simulink model "x35BusNetworkElectricityTransmissionModel"  (R2023b)
settings: Solver=VariableStepAuto  StartTime=0.0  StopTime=0.8  RelTol=1e-3
model workspace (MAT data in the model file):
  Compensation_Ki = 30
  Compensation_Kp = 3
  DC_Ki = 400
  DC_Kp = 8
  F = 0.01
  Flux_min = 0.5
  Grid_Freq_PWM = 2700
  Grid_Ireg_Ki = 5
  Grid_Ireg_Kp = 0.83
  Grid_Ireg_lim = 1.1
  Grid_Modindex_Upper = 1.1
  Grid_conv_Imax = 0.8
  H = 0.685
  Idref_max = 0.9
  Iqref_Tc = 0.3
  Ki_Var = 0.05
  Ki_Vreg = 20
  Ksh = 1.1
  L_pu = 0.3
  Llr = 0.16
  Lls = 0.18
  Lm = 2.9
  Nb_wt = 6
  P_mech = 1080000
  Pitch_Ki = 0
  Pitch_Kp = 150
  Pitch_Max = 27
  Pitch_Tc = 0.01
  Pitch_rate = 10
  Q_Filt = 50
  R_pu = 0.003
  Rotor_Freq_PWM = 1620
  Rotor_Ireg_Ki = 8
  Rotor_Ireg_Kp = 0.6
  Rotor_Ireg_lim = 0.1
  Rotor_Modindex_Upper = 2
  Rr = 0.016
  Rs = 0.023
  T_set = 0.0001
  Tp = 5e-05
  Ts = 5e-06
  Var_C_Filt = 720000
  Var_reg_max = 1.1
  Var_reg_min = 0.9
  WT_Coeff = [0.645 116 0.4 5 21 0.00912 0.08 0.035]
  WT_H = 4.32
  WT_IGBTRon = 5.931
  WT_Param = [91.204 10143]
  Wind_Freq_Filt = 10000
  Wind_Freq_nom = 60
  Wind_P_nom = 1200000
  Wind_Rotor_V_nom = 1950
  Wind_V_nom = 500
  Zeta_Filt = 0.707106781187
  init = [-0.2 0 0 0 0 0 0 0]
  p = 3
  torque0 = 0.83
  v_Ki = 0.1
  v_Kp = 3.6
  v_Max = 1.2
  v_Min = 0.7
  v_T = 5
  vreg_max = 1
  wind_VDC_nom = 1150
  wt0 = 1.2
undefined symbols (not defined in the file): D1, D11, Delta, DiscIntNeverNeededParam, Ion, Lithium, P, Q
libraries: powerlib_extras x144, spsSeriesRLCBranchLib x67, spsLoadFlowBusLib x43, spsThreePhaseTransformerTwoWindingsLib x32, spsThreePhaseSeriesRLCLoadLib x31, spsThreePhaseVIMeasurementLib x26, simulink_extras x26, spsDistributedParametersLineLib x22, spsGenericPowerSystemStabilizerLib x20, spsSynchronousMachinepuStandardLib x10, spsExcitationSystemLib x10, spsHydraulicTurbineandGovernorLib x10
(part 2 of 16)

== system x35BusNetworkElectricityTransmissionModel/ 41.4 MW Wind Generation ==
  " 64 MVA 115KV :20KV Transformer " : spsThreePhaseTransformerTwoWindingsLib/Three-Phase Transformer (Two Windings)  Winding1Connection=Yg  Winding2Connection=Delta (D1)  CoreType=Three single-phase transformers  SetSaturation=off  Hysteresis=off  DataFile='hysteresis'  SetInitialFlux=off  Measurements=None  UNITS=pu  NominalPower=[ 64e6 , 60 ]  Winding1=[ 115e3 , 0.002 , 0.08 ]  Winding2=[ 20e3 , 0.002 , 0.08 ]  Rm=500  Lm=500  L0=0.5  Saturation=[ 0,0 ; 0.0024,1.2 ; 1.0,1.52 ]  InitialFluxes=[ 0.8 , -0.8 , 0.7 ]  BreakLoop=off  DiscreteSolver=Trapezoidal iterative  DataType=off  TransfoNumber=1
  " Tie to Ground Transformer " : spsThreePhaseTransformerTwoWindingsLib/Three-Phase Transformer (Two Windings)  Winding1Connection=Yn  Winding2Connection=Delta (D11)  CoreType=Three single-phase transformers  SetSaturation=off  Hysteresis=off  DataFile='hysteresis'  SetInitialFlux=off  Measurements=None  UNITS=pu  NominalPower=[ 5600e6 , 60 ]  Winding1=[ 13.8e3 , 0.002 , 0.08 ]  Winding2=[ 735e3 , 0.002 , 0.08 ]  Rm=500  Lm=500  L0=0.5  Saturation=[ 0,0 ; 0.0024,1.2 ; 1.0,1.52 ]  InitialFluxes=[ 0.8 , -0.8 , 0.7 ]  BreakLoop=off  DiscreteSolver=Trapezoidal iterative  DataType=off  TransfoNumber=1
  150 kVar : spsThreePhaseSeriesRLCLoadLib/Three-Phase Series RLC Load  LConnTagsString=A|B|C  Configuration=Y (grounded)  NominalVoltage=20e3  Vabc=[1e3 1e3 1e3]  Vabcp=[1e3 1e3 1e3]  NominalFrequency=60  UnbalancedPower=off  ActivePower=0  InductivePower=0  CapacitivePower=150e3  Pabc=[10e3 9e3 11e3]  QLabc=[100 90 110]  QCabc=[100 90 110]  Pabcp=[10e3 9e3 11e3]  QLabcp=[100 90 110]  QCabcp=[100 90 110]  Measurements=None  LoadType=constant Z
  3.3MVar : spsThreePhaseSeriesRLCLoadLib/Three-Phase Series RLC Load  LConnTagsString=A|B|C  Configuration=Y (grounded)  NominalVoltage=20e3  Vabc=[1e3 1e3 1e3]  Vabcp=[1e3 1e3 1e3]  NominalFrequency=60  UnbalancedPower=off  ActivePower=0  InductivePower=0  CapacitivePower=3.3e6  Pabc=[10e3 9e3 11e3]  QLabc=[100 90 110]  QCabc=[100 90 110]  Pabcp=[10e3 9e3 11e3]  QLabcp=[100 90 110]  QCabcp=[100 90 110]  Measurements=None  LoadType=constant Z
  38 km : spsThreePhasePISectionLineLib/Three-Phase PI Section Line  LConnTagsString=a|b|c  RConnTagsString=A|B|C  Length=38  Frequency=60  Resistances=[ 0.01273 0.3864]/6  Inductances="[ 0.9337e-3  4.1264e-3]/6"  Capacitances=[12.74e-9 7.751e-9]*6
  41.4 MW Wind Farm : Subsystem
  4200 MW : spsThreePhaseParallelRLCLoadLib/Three-Phase Parallel RLC Load  LConnTagsString=A|B|C  Configuration=Y (grounded)  NominalVoltage=115e3  Vabc=[1e3 1e3 1e3]  Vabcp=[1e3 1e3 1e3]  NominalFrequency=60  UnbalancedPower=off  ActivePower=4200e6  InductivePower=0  CapacitivePower=0  Pabc=[10e3 9e3 11e3]  QLabc=[100 90 110]  QCabc=[100 90 110]  Pabcp=[10e3 9e3 11e3]  QLabcp=[100 90 110]  QCabcp=[100 90 110]  Measurements=None  LoadType=constant Z
  "4700 MVA 650KV :115KV Transformer " : spsThreePhaseTransformerTwoWindingsLib/Three-Phase Transformer (Two Windings)  Winding1Connection=Yg  Winding2Connection=Delta (D1)  CoreType=Three single-phase transformers  SetSaturation=off  Hysteresis=off  DataFile='hysteresis'  SetInitialFlux=off  Measurements=None  UNITS=pu  NominalPower=[ 4700e6 , 60 ]  Winding1=[ 650e3 , 0.002 , 0.08 ]  Winding2=[ 115e3 , 0.002 , 0.08 ]  Rm=500  Lm=500  L0=0.5  Saturation=[ 0,0 ; 0.0024,1.2 ; 1.0,1.52 ]  InitialFluxes=[ 0.8 , -0.8 , 0.7 ]  BreakLoop=off  DiscreteSolver=Trapezoidal iterative  DataType=off  TransfoNumber=1
  B2 : spsThreePhaseVIMeasurementLib/Three-Phase V-I Measurement  VoltageMeasurement=no  SetLabelV=off  LabelV=Vabc  Vpu=off  VpuLL=off  CurrentMeasurement=no  SetLabelI=off  LabelI=Iabc  Ipu=off  Pbase=100e6  Vbase=500e3  OutputType=Complex  PhasorSimulation=off  PSBequivalent=0
  Ground : spsGroundLib/Ground  LConnTagsString=a
  Load Flow Bus2 : spsLoadFlowBusLib/Load Flow Bus  LConnTagsString=a  Phases=single  Connectors=on one side  ID=BUS_28  Vbase=115e3  Vref=1  Vangle=0  VLF=1  VLFb=1  VLFc=1  angleLF=0  angleLFb=0  angleLFc=0
  Load Flow Bus7 : spsLoadFlowBusLib/Load Flow Bus  LConnTagsString=a  Phases=single  Connectors=on one side  ID=BUS_29  Vbase=20e3  Vref=1  Vangle=0  VLF=1  VLFb=1  VLFc=1  angleLF=0  angleLFb=0  angleLFc=0
  Series RLC Branch : spsSeriesRLCBranchLib/Series RLC Branch  LConnTagsString=__new0  RConnTagsString=__new0  BranchType=R  Resistance=4.1  Inductance=0  SetiL0=off  InitialCurrent=0  Capacitance=0  Setx0=off  InitialVoltage=0  Measurements=None
  A : PMIOPort  Side=Left
  B : PMIOPort  Port=2  Side=Left
  C : PMIOPort  Port=3  Side=Left
  connections:
  " Tie to Ground Transformer "/LConn4 -- Series RLC Branch/LConn1
  "4700 MVA 650KV :115KV Transformer "/RConn1 -- " 64 MVA 115KV :20KV Transformer "/LConn1 -- Load Flow Bus2/LConn1 -- 4200 MW/LConn1
  "4700 MVA 650KV :115KV Transformer "/RConn2 -- " 64 MVA 115KV :20KV Transformer "/LConn2 -- 4200 MW/LConn2
  "4700 MVA 650KV :115KV Transformer "/RConn3 -- " 64 MVA 115KV :20KV Transformer "/LConn3 -- 4200 MW/LConn3
  38 km/LConn2 -- " Tie to Ground Transformer "/LConn2 -- " 64 MVA 115KV :20KV Transformer "/RConn2 -- 3.3MVar/LConn2
  38 km/LConn3 -- " Tie to Ground Transformer "/LConn3 -- " 64 MVA 115KV :20KV Transformer "/RConn3 -- 3.3MVar/LConn3
  38 km/LConn1 -- " Tie to Ground Transformer "/LConn1 -- " 64 MVA 115KV :20KV Transformer "/RConn1 -- 3.3MVar/LConn1 -- Load Flow Bus7/LConn1
  Series RLC Branch/RConn1 -- Ground/LConn1
  "4700 MVA 650KV :115KV Transformer "/LConn1 -- A/RConn1
  "4700 MVA 650KV :115KV Transformer "/LConn3 -- C/RConn1
  "4700 MVA 650KV :115KV Transformer "/LConn2 -- B/RConn1
  150 kVar/LConn1 -- 38 km/RConn1 -- B2/RConn1
  B2/RConn3 -- 38 km/RConn3 -- 150 kVar/LConn3
  B2/RConn2 -- 38 km/RConn2 -- 150 kVar/LConn2
  41.4 MW Wind Farm/LConn1 -- B2/LConn1
  41.4 MW Wind Farm/LConn2 -- B2/LConn2
  41.4 MW Wind Farm/LConn3 -- B2/LConn3

== system x35BusNetworkElectricityTransmissionModel/400 kV Solar Farm ==
  3-Level Bridge : spsThreeLevelBridgeLib/Three-Level Bridge  Arms=3  SnubberResistance=1e6  SbubberCapacitance=inf  Device=IGBT / Diodes  Ron=0.2e-3  ForwardVoltages="[  0  0 ]"  Measurements=None
      settings: AttributesFormatString=\n
  "400 kVA 260V :25 kV Transformer " : spsThreePhaseTransformerTwoWindingsLib/Three-Phase Transformer (Two Windings)  Winding1Connection=Delta (D1)  Winding2Connection=Yg  CoreType=Three single-phase transformers  SetSaturation=off  Hysteresis=off  DataFile='hysteresis'  SetInitialFlux=off  Measurements=None  UNITS=pu  NominalPower=[ 400e3 , 60 ]  Winding1=[ 260 , 0.002 , 0.08 ]  Winding2=[ 25e3 , 0.002 , 0.08 ]  Rm=500  Lm=500  L0=0.5  Saturation=[ 0,0 ; 0.0024,1.2 ; 1.0,1.52 ]  InitialFluxes=[ 0.8 , -0.8 , 0.7 ]  BreakLoop=off  DiscreteSolver=Trapezoidal iterative  DataType=off  TransfoNumber=1
  "50 MVA 25kV :150 kV Transformer " : spsThreePhaseTransformerTwoWindingsLib/Three-Phase Transformer (Two Windings)  Winding1Connection=Delta (D1)  Winding2Connection=Yg  CoreType=Three single-phase transformers  SetSaturation=off  Hysteresis=off  DataFile='hysteresis'  SetInitialFlux=off  Measurements=None  UNITS=pu  NominalPower=[ 50e6 , 60 ]  Winding1=[ 25e3 , 0.002 , 0.08 ]  Winding2=[ 150e3 , 0.002 , 0.08 ]  Rm=500  Lm=500  L0=0.5  Saturation=[ 0,0 ; 0.0024,1.2 ; 1.0,1.52 ]  InitialFluxes=[ 0.8 , -0.8 , 0.7 ]  BreakLoop=off  DiscreteSolver=Trapezoidal iterative  DataType=off  TransfoNumber=1
  8000 MVA 150kV :650 kV Transformer 1 : spsThreePhaseTransformerTwoWindingsLib/Three-Phase Transformer (Two Windings)  Winding1Connection=Delta (D1)  Winding2Connection=Yg  CoreType=Three single-phase transformers  SetSaturation=off  Hysteresis=off  DataFile='hysteresis'  SetInitialFlux=off  Measurements=None  UNITS=pu  NominalPower=[8000e6 , 60 ]  Winding1=[ 150e3 , 0.002 , 0.08 ]  Winding2=[ 650e3 , 0.002 , 0.08 ]  Rm=500  Lm=500  L0=0.5  Saturation=[ 0,0 ; 0.0024,1.2 ; 1.0,1.52 ]  InitialFluxes=[ 0.8 , -0.8 , 0.7 ]  BreakLoop=off  DiscreteSolver=Trapezoidal iterative  DataType=off  TransfoNumber=1
  DC/DC Boost Converter : Subsystem
  DC/DC Boost Converter1 : Subsystem
  DC/DC Boost Converter2 : Subsystem
  DC/DC Boost Converter3 : Subsystem
  Deblock Converter : Step  Time=0.02  SampleTime=0
  Irradiance{,1..2,4} (4 alike) : eeStairGenerator/Stair Generator  LabelModeActiveChoice=Discrete  TimeInput=[0, 0.3, 0.5]  AmplitudeInput=[1000 100 1000]  SampleTime=Tp  RepeatPattern=off  OutDataTypeStr=double
      settings: LibrarySourceBlock=ee_sl_lib/General Control/Stair Generator
  Load Flow Bus1 : spsLoadFlowBusLib/Load Flow Bus  LConnTagsString=a  Phases=single  Connectors=on one side  ID=BUS_39  Vbase=25e3  Vref=1  Vangle=0  VLF=1  VLFb=1  VLFc=1  angleLF=0  angleLFb=0  angleLFc=0
  Load Flow Bus2 : spsLoadFlowBusLib/Load Flow Bus  LConnTagsString=a  Phases=single  Connectors=on one side  ID=BUS_40  Vbase=260  Vref=1  Vangle=0  VLF=1  VLFb=1  VLFc=1  angleLF=0  angleLFb=0  angleLFc=0
  Load Flow Bus6 : spsLoadFlowBusLib/Load Flow Bus  LConnTagsString=a  Phases=single  Connectors=on one side  ID=BUS_38  Vbase=150e3  Vref=1  Vangle=0  VLF=1  VLFb=1  VLFc=1  angleLF=0  angleLFb=0  angleLFc=0
  PV Array{,1..3} (4 alike) : spsPVArrayLib/PV Array  Npar=64  Nser=5  PlotType=array @ 1000 W/m2 & specified temperatures  S_vec="[ 1000  500  100 ]"  Temp_C_vec="[ 45 25  ]"  ModuleName=SunPower SPR-315E-WHT-D  PlotWhenSelected=off  Pm=315.072  Ncell=96  Voc=64.6  Isc=6.14  Vm=54.7  Im=5.76  beta_Voc_pc=-0.2727  alpha_Isc_pc=0.061743  beta_Voc=-0.17616  alpha_Isc=0.003791  IL=6.1461  I0=6.5067e-12  nI=0.95071  Rsh=430.0666  Rs=0.43041  RobustModel=on  RobustCellTemperature=45  BAL=on  Tc=1e-6  Tfilter=5e-5
  Product1 : Product
  Rate Limiter{,1..3} (4 alike) : RateLimiter  RisingSlewLimit=8000  FallingSlewLimit=-8000  SampleTimeMode=inherited  InitialCondition=1000
  Series RLC Branch1 : spsSeriesRLCBranchLib/Series RLC Branch  LConnTagsString=__new0  RConnTagsString=__new0  BranchType=C  Resistance=1  Inductance=1e-3  SetiL0=off  InitialCurrent=0  Capacitance=0.012  Setx0=off  InitialVoltage=250  Measurements=None
  Series RLC Branch2 : spsSeriesRLCBranchLib/Series RLC Branch  LConnTagsString=__new0  RConnTagsString=__new0  BranchType=C  Resistance=1  Inductance=1e-3  SetiL0=off  InitialCurrent=0  Capacitance=0.012  Setx0=off  InitialVoltage=250  Measurements=None
  Three-Phase Series RLC Branch : spsThreePhaseSeriesRLCBranchLib/Three-Phase Series RLC Branch  LConnTagsString=A|B|C  RConnTagsString=A|B|C  BranchType=RL  Resistance=1.2e-3  Inductance=45e-6  Capacitance=1e-6  Measurements=None
  Three-Phase Series RLC Load : spsThreePhaseSeriesRLCLoadLib/Three-Phase Series RLC Load  LConnTagsString=A|B|C  Configuration=Y (grounded)  NominalVoltage=260  Vabc=[1e3 1e3 1e3]  Vabcp=[1e3 1e3 1e3]  NominalFrequency=60  UnbalancedPower=off  ActivePower=41e3  InductivePower=0  CapacitivePower=41e3  Pabc=[10e3 9e3 11e3]  QLabc=[100 90 110]  QCabc=[100 90 110]  Pabcp=[10e3 9e3 11e3]  QLabcp=[100 90 110]  QCabcp=[100 90 110]  Measurements=None  LoadType=constant Z
  Three-Phase V-I Measurement1 : spsThreePhaseVIMeasurementLib/Three-Phase V-I Measurement  VoltageMeasurement=phase-to-ground  SetLabelV=on  LabelV=V_grid  Vpu=off  VpuLL=off  CurrentMeasurement=yes  SetLabelI=on  LabelI=I_grid  Ipu=off  Pbase=100e6  Vbase=500e3  OutputType=Complex  PhasorSimulation=off  PSBequivalent=0
  VSC Control : Subsystem  mask(VSC Main Controller){nom=[ 400e3  60 ], Vnom=[ 25e3 260 ], Vnom_dc=500, RLxfo=[0.002  0.06 ], RLchoke=[1e-3  45e-6  ], K_VDCreg=[7  800], K_Ireg=[0.3 20], Ts=T_set}
      mask prompts: nom "Nominal power and frequency [ Pnom(VA)  Fnom(Hz) ]:"; Vnom "Nominal primary and secondary voltages (Vrms LL) [ Vnom_prim   Vnom_sec ]:"; Vnom_dc "Nominal DC bus voltage (V):"; RLxfo "Total transformer leakage impedance (pu/Pnom) [ Rxfo  Lxf ]"; RLchoke "Choke impedance [ R(ohm) L(H) ]"; K_VDCreg "VDC regultator gains [ Kp  Ki ]:"; K_Ireg "Current regulator gains [ Kp  Ki ]:"; Ts "Sample time"
      mask init:
      | Pnom=nom(1);
      | Fnom=nom(2);
      | Vnom_prim=Vnom(1);
      | Vnom_sec=Vnom(2);
      | Zbase=Vnom_sec^2/Pnom;
      | Rtot_pu=RLxfo(1) + RLchoke(1)/Zbase;
      | Ltot_pu=RLxfo(2) + RLchoke(2)/(Zbase/(2*pi*Fnom));
      | Kp_VDCreg=K_VDCreg(1);
      | Ki_VDCreg=K_VDCreg(2);
      | Kp_Ireg=K_Ireg(1);
      | Ki_Ireg=K_Ireg(2);
      | Vdc_ref=Vnom_dc;
      | % Used to determine initial value of Boost Control (MPPT)
      | assignin('base','Vdc_ref_Inv',Vdc_ref);
  Voltage Measurement1 : spsVoltageMeasurementLib/Voltage Measurement  PhasorSimulation=off  OutputType=Complex  PSBequivalent=0
  A : PMIOPort  Side=Left
  "B " : PMIOPort  Port=2  Side=Left
  C : PMIOPort  Port=3  Side=Left
  wires:
  PV Array/1 -> DC/DC Boost Converter/1(m)
  Irradiance/1 -> Rate Limiter/1
  VSC Control/1(Pulses) -> Product1/2
  Product1/1 -> 3-Level Bridge/1
  Voltage Measurement1/1 -> [V_DC]
  [V_DC] -> VSC Control/3(Vdc_mes)
  [V_grid] -> VSC Control/1(Vabc_prim)
  [I_grid] -> VSC Control/2(Iabc_prim)
  PV Array1/1 -> DC/DC Boost Converter1/1(m)
  Irradiance4/1 -> Rate Limiter1/1
  PV Array2/1 -> DC/DC Boost Converter2/1(m)
  Irradiance1/1 -> Rate Limiter2/1
  Deblock Converter/1 -> Product1/1
  PV Array3/1 -> DC/DC Boost Converter3/1(m)
  Irradiance2/1 -> Rate Limiter3/1
  Rate Limiter/1 -> PV Array/1
  Rate Limiter1/1 -> PV Array1/1
  Rate Limiter2/1 -> PV Array2/1
  Rate Limiter3/1 -> PV Array3/1
  connections:
  Three-Phase Series RLC Load/LConn1 -- Three-Phase Series RLC Branch/RConn1 -- Load Flow Bus2/LConn1 -- "400 kVA 260V :25 kV Transformer "/LConn1
  Three-Phase Series RLC Load/LConn2 -- Three-Phase Series RLC Branch/RConn2 -- "400 kVA 260V :25 kV Transformer "/LConn2
  Three-Phase Series RLC Load/LConn3 -- Three-Phase Series RLC Branch/RConn3 -- "400 kVA 260V :25 kV Transformer "/LConn3
  8000 MVA 150kV :650 kV Transformer 1/LConn1 -- "50 MVA 25kV :150 kV Transformer "/RConn1 -- Load Flow Bus6/LConn1
  8000 MVA 150kV :650 kV Transformer 1/LConn2 -- "50 MVA 25kV :150 kV Transformer "/RConn2
  "50 MVA 25kV :150 kV Transformer "/RConn3 -- 8000 MVA 150kV :650 kV Transformer 1/LConn3
  A/RConn1 -- 8000 MVA 150kV :650 kV Transformer 1/RConn1
  "B "/RConn1 -- 8000 MVA 150kV :650 kV Transformer 1/RConn2
  C/RConn1 -- 8000 MVA 150kV :650 kV Transformer 1/RConn3
  Three-Phase Series RLC Branch/LConn1 -- 3-Level Bridge/LConn1
  Three-Phase Series RLC Branch/LConn2 -- 3-Level Bridge/LConn2
  Three-Phase Series RLC Branch/LConn3 -- 3-Level Bridge/LConn3
  DC/DC Boost Converter/LConn1 -- PV Array/RConn1
  DC/DC Boost Converter/LConn2 -- PV Array/RConn2
  DC/DC Boost Converter1/LConn2 -- PV Array1/RConn2
  DC/DC Boost Converter1/LConn1 -- PV Array1/RConn1
  DC/DC Boost Converter2/LConn2 -- PV Array2/RConn2
  DC/DC Boost Converter2/LConn1 -- PV Array2/RConn1
  Series RLC Branch1/RConn1 -- Series RLC Branch2/LConn1 -- 3-Level Bridge/RConn2
  DC/DC Boost Converter/RConn1 -- Voltage Measurement1/LConn1 -- 3-Level Bridge/RConn1 -- Series RLC Branch1/LConn1 -- DC/DC Boost Converter1/RConn1 -- DC/DC Boost Converter3/RConn1 -- DC/DC Boost Converter2/RConn1
  DC/DC Boost Converter/RConn2 -- DC/DC Boost Converter1/RConn2 -- 3-Level Bridge/RConn3 -- Voltage Measurement1/LConn2 -- Series RLC Branch2/RConn1 -- DC/DC Boost Converter3/RConn2 -- DC/DC Boost Converter2/RConn2
  DC/DC Boost Converter3/LConn1 -- PV Array3/RConn1
  DC/DC Boost Converter3/LConn2 -- PV Array3/RConn2
  Three-Phase V-I Measurement1/LConn1 -- "400 kVA 260V :25 kV Transformer "/RConn1
  Three-Phase V-I Measurement1/LConn2 -- "400 kVA 260V :25 kV Transformer "/RConn2
  Three-Phase V-I Measurement1/LConn3 -- "400 kVA 260V :25 kV Transformer "/RConn3
  Three-Phase V-I Measurement1/RConn3 -- "50 MVA 25kV :150 kV Transformer "/LConn3
  Three-Phase V-I Measurement1/RConn2 -- "50 MVA 25kV :150 kV Transformer "/LConn2
  Three-Phase V-I Measurement1/RConn1 -- "50 MVA 25kV :150 kV Transformer "/LConn1 -- Load Flow Bus1/LConn1

== system x35BusNetworkElectricityTransmissionModel/BESS ==
  "45 MVA 20kV :250 kV Transformer " : spsThreePhaseTransformerTwoWindingsLib/Three-Phase Transformer (Two Windings)  Winding1Connection=Delta (D1)  Winding2Connection=Yg  CoreType=Three single-phase transformers  SetSaturation=off  Hysteresis=off  DataFile='hysteresis'  SetInitialFlux=off  Measurements=None  UNITS=pu  NominalPower=[ 45e6 , 60 ]  Winding1=[ 20e3 , 0.002 , 0.08 ]  Winding2=[ 250e3 , 0.002 , 0.08 ]  Rm=500  Lm=500  L0=0.5  Saturation=[ 0,0 ; 0.0024,1.2 ; 1.0,1.52 ]  InitialFluxes=[ 0.8 , -0.8 , 0.7 ]  BreakLoop=off  DiscreteSolver=Trapezoidal iterative  DataType=off  TransfoNumber=1
  "450 kVA 250 V :20 kV Transformer " : spsThreePhaseTransformerTwoWindingsLib/Three-Phase Transformer (Two Windings)  Winding1Connection=Delta (D1)  Winding2Connection=Yg  CoreType=Three single-phase transformers  SetSaturation=off  Hysteresis=off  DataFile='hysteresis'  SetInitialFlux=off  Measurements=None  UNITS=pu  NominalPower=[ 450e3 , 60 ]  Winding1=[ 250 , 0.002 , 0.08 ]  Winding2=[ 20e3 , 0.002 , 0.08 ]  Rm=500  Lm=500  L0=0.5  Saturation=[ 0,0 ; 0.0024,1.2 ; 1.0,1.52 ]  InitialFluxes=[ 0.8 , -0.8 , 0.7 ]  BreakLoop=off  DiscreteSolver=Trapezoidal iterative  DataType=off  TransfoNumber=1
  "5000 MVA 250kV :650 kV Transformer " : spsThreePhaseTransformerTwoWindingsLib/Three-Phase Transformer (Two Windings)  Winding1Connection=Delta (D1)  Winding2Connection=Yg  CoreType=Three single-phase transformers  SetSaturation=off  Hysteresis=off  DataFile='hysteresis'  SetInitialFlux=off  Measurements=None  UNITS=pu  NominalPower=[ 5000e6 , 60 ]  Winding1=[ 250e3 , 0.002 , 0.08 ]  Winding2=[ 650e3 , 0.002 , 0.08 ]  Rm=500  Lm=500  L0=0.5  Saturation=[ 0,0 ; 0.0024,1.2 ; 1.0,1.52 ]  InitialFluxes=[ 0.8 , -0.8 , 0.7 ]  BreakLoop=off  DiscreteSolver=Trapezoidal iterative  DataType=off  TransfoNumber=1
  Battery Management System : Subsystem
  Battery2 : spsBatteryLib/Battery  BatType=Lithium-Ion  ShowTempParam=off  ThermalPreset=no  ShowAgeParam=off  NomV=250  NomQ=3e5  SOC=95  Batt_Tr=30  PresetModel=on  MaxQ=300000  MinV=187.5  FullV=290.9968  Dis_rate=130434.7826  R=8.3333e-06  Normal_OP=271304.3478  expZone="[270.096463      14739.1304]"  current=[6.5 13 32.5]  Units=Time  Tci=20  NomT=20  T2=-30  MaxQ2=4.8  FullV2=7.1  Normal_OP2=5.655  expZone2="[6.58           1]"  Rca=0.6  ti=2000  Dp=0  Neq0=0  Tsim=1e6  Ta1=25  Qeol=5.4*0.9  Reol=0.013333*1.2  Char_age=[2.3478, 3]  Dis_age=[2.3478, 10]  N1=1500  N2=10500  N3=1000  N4=1400  Ta2=45  N5=950
  Bus Selector : BusSelector  OutputSignals=SOC (%),Current (A),Voltage (V)
  IGBT/Diode : spsIGBTDiodeLib/IGBT//Diode  Ron=1e-3  Rs=1e5  Cs=inf  Measurements=on
  IGBT/Diode1 : spsIGBTDiodeLib/IGBT//Diode  Ron=1e-3  Rs=1e5  Cs=inf  Measurements=on
  Power Calculation : Subsystem
  Series RLC Branch : spsSeriesRLCBranchLib/Series RLC Branch  LConnTagsString=__new0  RConnTagsString=__new0  BranchType=L  Resistance=0  Inductance=2e-3  SetiL0=off  InitialCurrent=0  Capacitance=0  Setx0=off  InitialVoltage=0  Measurements=None
  Series RLC Branch3 : spsSeriesRLCBranchLib/Series RLC Branch  LConnTagsString=__new0  RConnTagsString=__new0  BranchType=RL  Resistance=0.058  Inductance=20  SetiL0=off  InitialCurrent=0  Capacitance=1e-6  Setx0=off  InitialVoltage=0  Measurements=None
  Series RLC Branch4 : spsSeriesRLCBranchLib/Series RLC Branch  LConnTagsString=__new0  RConnTagsString=__new0  BranchType=R  Resistance=2  Inductance=20  SetiL0=off  InitialCurrent=0  Capacitance=1e-6  Setx0=off  InitialVoltage=0  Measurements=None
  Terminator : Terminator
  Terminator1 : Terminator
  Three-Phase Breaker : spsThreePhaseBreakerLib/Three-Phase Breaker  InitialState=open  SwitchA=on  SwitchB=on  SwitchC=on  SwitchTimes="[0.2  0.5]"  External=off  BreakerResistance=0.01  SnubberResistance=1e6  SnubberCapacitance=inf  Measurements=None
  Universal Bridge : spsUniversalBridgeLib/Universal Bridge  Arms=3  SnubberResistance=1e5  SnubberCapacitance=inf  Device=Diodes  Ron=1e-3  Lon=0  ForwardVoltages="[  0  0  ]"  ForwardVoltage=0  GTOparameters=[ 10e-6 , 20e-6 ]  IGBTparameters=[ 1e-6 , 2e-6 ]  Measurements=None  Measurements_2=None  converterType=Rectifier
  Voltage Measurement : spsVoltageMeasurementLib/Voltage Measurement  PhasorSimulation=off  OutputType=Complex  PSBequivalent=0
  A : PMIOPort  Side=Left
  B : PMIOPort  Port=2  Side=Left
  C : PMIOPort  Port=3  Side=Left
  tag scope: BESS_Iabc=global, BESS_Vabc=global, SOC=global
  wires:
  [S_PES] -> IGBT/Diode1/1
  Bus Selector/1 -> [SOC]  "<SOC (%)>"
  Voltage Measurement/1 -> [BESS_VDC]
  [S_NES] -> IGBT/Diode/1
  Battery2/1 -> Bus Selector/1
  Bus Selector/3 -> [BESS_Vabc]  "<Voltage (V)>"
  Bus Selector/2 -> [BESS_Iabc]  "<Current (A)>"
  IGBT/Diode1/1 -> Terminator/1
  IGBT/Diode/1 -> Terminator1/1
  connections:
  Series RLC Branch4/RConn1 -- Series RLC Branch3/RConn1 -- IGBT/Diode/RConn1 -- Battery2/LConn2 -- Voltage Measurement/LConn2 -- Universal Bridge/RConn2
  Series RLC Branch4/LConn1 -- Series RLC Branch3/LConn1 -- IGBT/Diode1/RConn1 -- Voltage Measurement/LConn1 -- Universal Bridge/RConn1
  Series RLC Branch/LConn1 -- Battery2/LConn1
  Series RLC Branch/RConn1 -- IGBT/Diode/LConn1 -- IGBT/Diode1/LConn1
  Universal Bridge/LConn1 -- Three-Phase Breaker/LConn1
  Universal Bridge/LConn2 -- Three-Phase Breaker/LConn2
  Universal Bridge/LConn3 -- Three-Phase Breaker/LConn3
  "450 kVA 250 V :20 kV Transformer "/LConn1 -- Three-Phase Breaker/RConn1
  "450 kVA 250 V :20 kV Transformer "/LConn2 -- Three-Phase Breaker/RConn2
  "450 kVA 250 V :20 kV Transformer "/LConn3 -- Three-Phase Breaker/RConn3
  "45 MVA 20kV :250 kV Transformer "/LConn1 -- "450 kVA 250 V :20 kV Transformer "/RConn1
  "450 kVA 250 V :20 kV Transformer "/RConn2 -- "45 MVA 20kV :250 kV Transformer "/LConn2
  "450 kVA 250 V :20 kV Transformer "/RConn3 -- "45 MVA 20kV :250 kV Transformer "/LConn3
  "5000 MVA 250kV :650 kV Transformer "/LConn1 -- "45 MVA 20kV :250 kV Transformer "/RConn1
  "5000 MVA 250kV :650 kV Transformer "/LConn2 -- "45 MVA 20kV :250 kV Transformer "/RConn2
  "5000 MVA 250kV :650 kV Transformer "/LConn3 -- "45 MVA 20kV :250 kV Transformer "/RConn3
  "5000 MVA 250kV :650 kV Transformer "/RConn3 -- C/RConn1
  B/RConn1 -- "5000 MVA 250kV :650 kV Transformer "/RConn2
  A/RConn1 -- "5000 MVA 250kV :650 kV Transformer "/RConn1

== system x35BusNetworkElectricityTransmissionModel/Cs MPOD ==
  Series RLC Branch : spsSeriesRLCBranchLib/Series RLC Branch  LConnTagsString=__new0  RConnTagsString=__new0  BranchType=C  Resistance=1  Inductance=1e-3  SetiL0=off  InitialCurrent=0  Capacitance=0.00049736  Setx0=off  InitialVoltage=0  Measurements=None
  Series RLC Branch1 : spsSeriesRLCBranchLib/Series RLC Branch  LConnTagsString=__new0  RConnTagsString=__new0  BranchType=C  Resistance=1  Inductance=1e-3  SetiL0=off  InitialCurrent=0  Capacitance=0.00049736  Setx0=off  InitialVoltage=0  Measurements=None
  Series RLC Branch2 : spsSeriesRLCBranchLib/Series RLC Branch  LConnTagsString=__new0  RConnTagsString=__new0  BranchType=C  Resistance=1  Inductance=1e-3  SetiL0=off  InitialCurrent=0  Capacitance=0.00049736  Setx0=off  InitialVoltage=0  Measurements=None
  A : PMIOPort  Side=Left
  A1 : PMIOPort  Port=2  Side=Right
  B : PMIOPort  Port=3  Side=Left
  B1 : PMIOPort  Port=4  Side=Right
  C : PMIOPort  Port=5  Side=Left
  C1 : PMIOPort  Port=6  Side=Right
  connections:
  A1/RConn1 -- Series RLC Branch/RConn1
  B1/RConn1 -- Series RLC Branch1/RConn1
  A/RConn1 -- Series RLC Branch/LConn1
  C/RConn1 -- Series RLC Branch2/LConn1
  B/RConn1 -- Series RLC Branch1/LConn1
  C1/RConn1 -- Series RLC Branch2/RConn1

== system x35BusNetworkElectricityTransmissionModel/Cs OSIS ==
  Series RLC Branch : spsSeriesRLCBranchLib/Series RLC Branch  LConnTagsString=__new0  RConnTagsString=__new0  BranchType=C  Resistance=1  Inductance=1e-3  SetiL0=off  InitialCurrent=0  Capacitance=0.00049736  Setx0=off  InitialVoltage=0  Measurements=None
  Series RLC Branch1 : spsSeriesRLCBranchLib/Series RLC Branch  LConnTagsString=__new0  RConnTagsString=__new0  BranchType=C  Resistance=1  Inductance=1e-3  SetiL0=off  InitialCurrent=0  Capacitance=0.00049736  Setx0=off  InitialVoltage=0  Measurements=None
  Series RLC Branch2 : spsSeriesRLCBranchLib/Series RLC Branch  LConnTagsString=__new0  RConnTagsString=__new0  BranchType=C  Resistance=1  Inductance=1e-3  SetiL0=off  InitialCurrent=0  Capacitance=0.00049736  Setx0=off  InitialVoltage=0  Measurements=None
  A : PMIOPort  Side=Left
  A1 : PMIOPort  Port=2  Side=Right
  B : PMIOPort  Port=3  Side=Left
  B1 : PMIOPort  Port=4  Side=Right
  C : PMIOPort  Port=5  Side=Left
  C1 : PMIOPort  Port=6  Side=Right
  connections:
  A1/RConn1 -- Series RLC Branch/RConn1
  B1/RConn1 -- Series RLC Branch1/RConn1
  A/RConn1 -- Series RLC Branch/LConn1
  C/RConn1 -- Series RLC Branch2/LConn1
  B/RConn1 -- Series RLC Branch1/LConn1
  C1/RConn1 -- Series RLC Branch2/RConn1

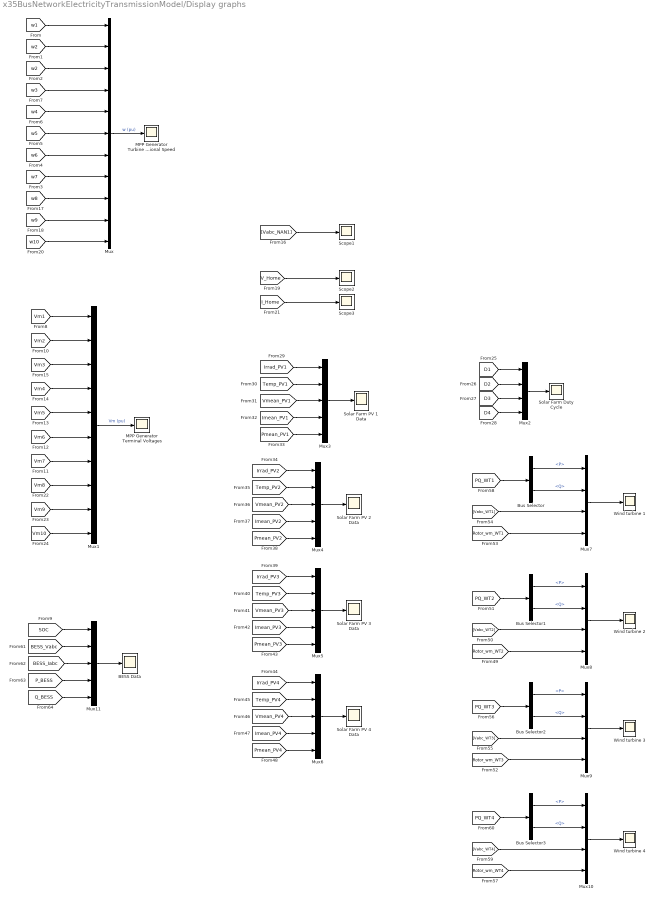
== system x35BusNetworkElectricityTransmissionModel/Display graphs ==
  BESS Data : Scope
  Bus Selector{,1..3} (4 alike) : BusSelector  OutputSignals=P,Q
  MPP Generator Terminal Voltages : Scope
  MPP Generator Turbine Rotational Speed : Scope
  Mux : Mux  Inputs=11
  Mux1 : Mux  Inputs=10
  Mux{2,7..10} (5 alike) : Mux
  Mux{3..6,11} (5 alike) : Mux  Inputs=5
  Scope1 : Scope
  Scope2 : Scope
  Scope3 : Scope
  Solar Farm Duty Cycle : Scope
  Solar Farm PV 1 Data : Scope
  Solar Farm PV 2 Data : Scope
  Solar Farm PV 3 Data : Scope
  Solar Farm PV 4 Data : Scope
  Wind turbine {1..4} (4 alike) : Scope
  wires:
  [w2] -> Mux/2
  [Vm5] -> Mux1/5
  [Vm3] -> Mux1/3
  [Vm1] -> Mux1/1
  [Vm4] -> Mux1/4
  [Vm6] -> Mux1/6
  [Vm2] -> Mux1/2
  [w6] -> Mux/7
  [Vm7] -> Mux1/7
  Mux1/1 -> MPP Generator Terminal Voltages/1  "Vm (pu)"
  [w2] -> Mux/3
  [w1] -> Mux/1
  [w3] -> Mux/4
  [w4] -> Mux/5
  [Vabc_NAN1] -> Scope1/1
  Mux/1 -> MPP Generator Turbine Rotational Speed/1  "w (pu)"
  [w7] -> Mux/8
  [w5] -> Mux/6
  [w8] -> Mux/9
  [w9] -> Mux/10
  [w10] -> Mux/11
  [V_Home] -> Scope2/1
  [I_Home] -> Scope3/1
  [Vm10] -> Mux1/10
  [Vm9] -> Mux1/9
  [Vm8] -> Mux1/8
  [D3] -> Mux2/3
  [D4] -> Mux2/4
  Mux2/1 -> Solar Farm Duty Cycle/1
  [D2] -> Mux2/2
  [D1] -> Mux2/1
  [Irrad_PV1] -> Mux3/1
  [Temp_PV1] -> Mux3/2
  [Vmean_PV1] -> Mux3/3
  [Imean_PV1] -> Mux3/4
  [Pmean_PV1] -> Mux3/5
  Mux3/1 -> Solar Farm PV 1 Data/1
  [Irrad_PV2] -> Mux4/1
  [Temp_PV2] -> Mux4/2
  Mux4/1 -> Solar Farm PV 2 Data/1
  [Imean_PV2] -> Mux4/4
  [Vmean_PV2] -> Mux4/3
  [Pmean_PV2] -> Mux4/5
  [Irrad_PV3] -> Mux5/1
  [Temp_PV3] -> Mux5/2
  Mux5/1 -> Solar Farm PV 3 Data/1
  [Imean_PV3] -> Mux5/4
  [Vmean_PV3] -> Mux5/3
  [Pmean_PV3] -> Mux5/5
  [Irrad_PV4] -> Mux6/1
  [Temp_PV4] -> Mux6/2
  Mux6/1 -> Solar Farm PV 4 Data/1
  [Imean_PV4] -> Mux6/4
  [Vmean_PV4] -> Mux6/3
  [Pmean_PV4] -> Mux6/5
  [Rotor_wm_WT1] -> Mux7/4
  [Vabc_WT1] -> Mux7/3
  Bus Selector/2 -> Mux7/2  "<Q>"
  [PQ_WT1] -> Bus Selector/1
  Bus Selector/1 -> Mux7/1  "<P>"
  Mux7/1 -> Wind turbine 1/1
  Bus Selector1/1 -> Mux8/1  "<P>"
  Mux8/1 -> Wind turbine 2/1
  [Rotor_wm_WT2] -> Mux8/4
  [PQ_WT2] -> Bus Selector1/1
  Bus Selector1/2 -> Mux8/2  "<Q>"
  [Vabc_WT2] -> Mux8/3
  Bus Selector2/1 -> Mux9/1  "<P>"
  Mux9/1 -> Wind turbine 3/1
  [Rotor_wm_WT3] -> Mux9/4
  [PQ_WT3] -> Bus Selector2/1
  Bus Selector2/2 -> Mux9/2  "<Q>"
  [Vabc_WT3] -> Mux9/3
  Bus Selector3/1 -> Mux10/1  "<P>"
  Mux10/1 -> Wind turbine 4/1
  [Rotor_wm_WT4] -> Mux10/4
  [PQ_WT4] -> Bus Selector3/1
  Bus Selector3/2 -> Mux10/2  "<Q>"
  [Vabc_WT4] -> Mux10/3
  [P_BESS] -> Mux11/4
  [Q_BESS] -> Mux11/5
  [BESS_Iabc] -> Mux11/3
  Mux11/1 -> BESS Data/1
  [BESS_Vabc] -> Mux11/2
  [SOC] -> Mux11/1

== system x35BusNetworkElectricityTransmissionModel/Home Network Load （with circuit breaker) ==
  " Refrigerator 120V 767W" : spsParallelRLCLoadLib/Parallel RLC Load  LConnTagsString=a  RConnTagsString=__new0  NominalVoltage=120  NominalFrequency=60  ActivePower=767  InductivePower=0  CapacitivePower=0  Setx0=off  InitialVoltage=0  SetiL0=off  InitialCurrent=0  Measurements=None  LoadType=constant Z
      settings: AttributesFormatString=\n  LibrarySourceBlock=sps_lib/Passives/Parallel RLC Load
  "14000 MVA 150KV :15KV Transformer " : spsThreePhaseTransformerTwoWindingsLib/Three-Phase Transformer (Two Windings)  Winding1Connection=Yg  Winding2Connection=Delta (D1)  CoreType=Three single-phase transformers  SetSaturation=off  Hysteresis=off  DataFile='hysteresis'  SetInitialFlux=off  Measurements=None  UNITS=pu  NominalPower=[ 14000e6 , 60 ]  Winding1=[ 150e3 , 0.002 , 0.08 ]  Winding2=[ 15e3 , 0.002 , 0.08 ]  Rm=500  Lm=500  L0=0.5  Saturation=[ 0,0 ; 0.0024,1.2 ; 1.0,1.52 ]  InitialFluxes=[ 0.8 , -0.8 , 0.7 ]  BreakLoop=off  DiscreteSolver=Trapezoidal iterative  DataType=off  TransfoNumber=1
  1700 Mvar : spsThreePhaseSeriesRLCLoadLib/Three-Phase Series RLC Load  LConnTagsString=A|B|C  Configuration=Y (grounded)  NominalVoltage=150e3  Vabc=[1e3 1e3 1e3]  Vabcp=[1e3 1e3 1e3]  NominalFrequency=60  UnbalancedPower=off  ActivePower=0  InductivePower=0  CapacitivePower=1700e6  Pabc=[10e3 9e3 11e3]  QLabc=[100 90 110]  QCabc=[100 90 110]  Pabcp=[10e3 9e3 11e3]  QLabcp=[100 90 110]  QCabcp=[100 90 110]  Measurements=None  LoadType=constant Z
  "18000 MVA 650KV :150KV Transformer " : spsThreePhaseTransformerTwoWindingsLib/Three-Phase Transformer (Two Windings)  Winding1Connection=Yg  Winding2Connection=Delta (D1)  CoreType=Three single-phase transformers  SetSaturation=off  Hysteresis=off  DataFile='hysteresis'  SetInitialFlux=off  Measurements=None  UNITS=pu  NominalPower=[ 18000e6 , 60 ]  Winding1=[ 650e3 , 0.002 , 0.08 ]  Winding2=[ 150e3 , 0.002 , 0.08 ]  Rm=500  Lm=500  L0=0.5  Saturation=[ 0,0 ; 0.0024,1.2 ; 1.0,1.52 ]  InitialFluxes=[ 0.8 , -0.8 , 0.7 ]  BreakLoop=off  DiscreteSolver=Trapezoidal iterative  DataType=off  TransfoNumber=1
  4 kW 150 V Load : spsParallelRLCLoadLib/Parallel RLC Load  LConnTagsString=a  RConnTagsString=__new0  NominalVoltage=150  NominalFrequency=60  ActivePower=4e3  InductivePower=100  CapacitivePower=100  Setx0=off  InitialVoltage=0  SetiL0=off  InitialCurrent=0  Measurements=None  LoadType=constant Z
      settings: AttributesFormatString=\n  LibrarySourceBlock=sps_lib/Passives/Parallel RLC Load
  "80 kVA 15KV :150 V Transformer " : spsThreePhaseTransformerTwoWindingsLib/Three-Phase Transformer (Two Windings)  Winding1Connection=Yg  Winding2Connection=Yg  CoreType=Three single-phase transformers  SetSaturation=off  Hysteresis=off  DataFile='hysteresis'  SetInitialFlux=off  Measurements=None  UNITS=pu  NominalPower=[ 80e3 , 60 ]  Winding1=[ 15e3 , 0.002 , 0.08 ]  Winding2=[ 150 , 0.002 , 0.08 ]  Rm=500  Lm=500  L0=0.5  Saturation=[ 0,0 ; 0.0024,1.2 ; 1.0,1.52 ]  InitialFluxes=[ 0.8 , -0.8 , 0.7 ]  BreakLoop=off  DiscreteSolver=Trapezoidal iterative  DataType=off  TransfoNumber=1
  Breaker1 : spsBreakerLib/Breaker  InitialState=0  SwitchingTimes=[.05 0.1]  External=off  BreakerResistance=1e-5  SnubberResistance=1e6  SnubberCapacitance=inf  Measurements=None  MoreParameters=off  NoBreakLoop=off
      settings: AttributesFormatString=\n
  Circuit Breaker : Subsystem
  Current Measurement : spsCurrentMeasurementLib/Current Measurement  PhasorSimulation=off  OutputType=Complex  PSBequivalent=0
  Ground : spsGroundLib/Ground  LConnTagsString=a
  Lamp 5V 30W : spsParallelRLCLoadLib/Parallel RLC Load  LConnTagsString=a  RConnTagsString=__new0  NominalVoltage=5  NominalFrequency=60  ActivePower=30  InductivePower=0  CapacitivePower=0  Setx0=off  InitialVoltage=0  SetiL0=off  InitialCurrent=0  Measurements=None  LoadType=constant Z
      settings: AttributesFormatString=\n  LibrarySourceBlock=sps_lib/Passives/Parallel RLC Load
  Load Flow Bus1 : spsLoadFlowBusLib/Load Flow Bus  LConnTagsString=a  Phases=single  Connectors=on one side  ID=BUS_41  Vbase=150e3  Vref=1  Vangle=0  VLF=1  VLFb=1  VLFc=1  angleLF=0  angleLFb=0  angleLFc=0
  Load Flow Bus2 : spsLoadFlowBusLib/Load Flow Bus  LConnTagsString=a  Phases=single  Connectors=on one side  ID=BUS_43  Vbase=150  Vref=1  Vangle=0  VLF=1  VLFb=1  VLFc=1  angleLF=0  angleLFb=0  angleLFc=0
  Load Flow Bus6 : spsLoadFlowBusLib/Load Flow Bus  LConnTagsString=a  Phases=single  Connectors=on one side  ID=BUS_42  Vbase=15e3  Vref=1  Vangle=0  VLF=1  VLFb=1  VLFc=1  angleLF=0  angleLFb=0  angleLFc=0
  Stair Generator : eeStairGenerator/Stair Generator  LabelModeActiveChoice=Continuous  TimeInput=[0 0.1 0.2]  AmplitudeInput=[0 1 0]  SampleTime=0  RepeatPattern=off  OutDataTypeStr=double
      settings: LibrarySourceBlock=ee_sl_lib/General Control/Stair Generator
  Three-Level Bridge : spsThreeLevelBridgeLib/Three-Level Bridge  Arms=3  SnubberResistance=1e5  SbubberCapacitance=inf  Device=GTO / Diodes  Ron=1e-3  ForwardVoltages="[  0  0  ]"  Measurements=None
      settings: LibrarySourceBlock=sps_lib/Power Electronics/Three-Level Bridge
  Voltage Measurement : spsVoltageMeasurementLib/Voltage Measurement  PhasorSimulation=off  OutputType=Complex  PSBequivalent=0
  A : PMIOPort  Side=Left
  B : PMIOPort  Port=2  Side=Left
  C : PMIOPort  Port=3  Side=Left
  tag scope: I_Home=global, V_Home=global
  wires:
  Stair Generator/1 -> Circuit Breaker/1("Reset ")
  Current Measurement/1 -> [I_Home]
  Voltage Measurement/1 -> [V_Home]
  connections:
  "18000 MVA 650KV :150KV Transformer "/RConn1 -- 1700 Mvar/LConn1 -- "14000 MVA 150KV :15KV Transformer "/LConn1 -- Load Flow Bus1/LConn1
  "18000 MVA 650KV :150KV Transformer "/LConn1 -- A/RConn1
  "18000 MVA 650KV :150KV Transformer "/RConn3 -- "14000 MVA 150KV :15KV Transformer "/LConn3 -- 1700 Mvar/LConn3
  "14000 MVA 150KV :15KV Transformer "/LConn2 -- "18000 MVA 650KV :150KV Transformer "/RConn2 -- 1700 Mvar/LConn2
  "18000 MVA 650KV :150KV Transformer "/LConn2 -- B/RConn1
  "18000 MVA 650KV :150KV Transformer "/LConn3 -- C/RConn1
  "14000 MVA 150KV :15KV Transformer "/RConn1 -- Load Flow Bus6/LConn1 -- "80 kVA 15KV :150 V Transformer "/LConn1
  "80 kVA 15KV :150 V Transformer "/LConn2 -- "14000 MVA 150KV :15KV Transformer "/RConn2
  "80 kVA 15KV :150 V Transformer "/LConn3 -- "14000 MVA 150KV :15KV Transformer "/RConn3
  "80 kVA 15KV :150 V Transformer "/RConn1 -- Load Flow Bus2/LConn1 -- Three-Level Bridge/LConn1
  "80 kVA 15KV :150 V Transformer "/RConn2 -- Three-Level Bridge/LConn2
  "80 kVA 15KV :150 V Transformer "/RConn3 -- Three-Level Bridge/LConn3
  Three-Level Bridge/RConn1 -- Current Measurement/LConn1 -- 4 kW 150 V Load/LConn1
  4 kW 150 V Load/RConn1 -- Lamp 5V 30W/RConn1 -- " Refrigerator 120V 767W"/RConn1 -- Three-Level Bridge/RConn3
  Voltage Measurement/LConn2 -- Breaker1/LConn1 -- " Refrigerator 120V 767W"/LConn1 -- Circuit Breaker/RConn1
  Ground/LConn1 -- Three-Level Bridge/RConn2
  Voltage Measurement/LConn1 -- Circuit Breaker/LConn1 -- Current Measurement/RConn1
  Lamp 5V 30W/LConn1 -- Breaker1/RConn1

== system x35BusNetworkElectricityTransmissionModel/MTL Load ==
  1.8 Mvar : spsThreePhaseSeriesRLCLoadLib/Three-Phase Series RLC Load  LConnTagsString=A|B|C  Configuration=Y (grounded)  NominalVoltage=20e3  Vabc=[1e3 1e3 1e3]  Vabcp=[1e3 1e3 1e3]  NominalFrequency=60  UnbalancedPower=off  ActivePower=0  InductivePower=0  CapacitivePower=1.8e6  Pabc=[10e3 9e3 11e3]  QLabc=[100 90 110]  QCabc=[100 90 110]  Pabcp=[10e3 9e3 11e3]  QLabcp=[100 90 110]  QCabcp=[100 90 110]  Measurements=None  LoadType=constant Z
  "15800 MVA 300KV :20KV Transformer " : spsThreePhaseTransformerTwoWindingsLib/Three-Phase Transformer (Two Windings)  Winding1Connection=Yg  Winding2Connection=Delta (D1)  CoreType=Three single-phase transformers  SetSaturation=off  Hysteresis=off  DataFile='hysteresis'  SetInitialFlux=off  Measurements=None  UNITS=pu  NominalPower=[ 15800e6 , 60 ]  Winding1=[ 300e3 , 0.002 , 0.08 ]  Winding2=[ 20e3 , 0.002 , 0.08 ]  Rm=500  Lm=500  L0=0.5  Saturation=[ 0,0 ; 0.0024,1.2 ; 1.0,1.52 ]  InitialFluxes=[ 0.8 , -0.8 , 0.7 ]  BreakLoop=off  DiscreteSolver=Trapezoidal iterative  DataType=off  TransfoNumber=1
  "19000 MVA 650KV :300KV Transformer " : spsThreePhaseTransformerTwoWindingsLib/Three-Phase Transformer (Two Windings)  Winding1Connection=Yg  Winding2Connection=Delta (D1)  CoreType=Three single-phase transformers  SetSaturation=off  Hysteresis=off  DataFile='hysteresis'  SetInitialFlux=off  Measurements=None  UNITS=pu  NominalPower=[ 19000e6 , 60 ]  Winding1=[ 650e3 , 0.002 , 0.08 ]  Winding2=[ 300e3 , 0.002 , 0.08 ]  Rm=500  Lm=500  L0=0.5  Saturation=[ 0,0 ; 0.0024,1.2 ; 1.0,1.52 ]  InitialFluxes=[ 0.8 , -0.8 , 0.7 ]  BreakLoop=off  DiscreteSolver=Trapezoidal iterative  DataType=off  TransfoNumber=1
  2800 Mvar : spsThreePhaseSeriesRLCLoadLib/Three-Phase Series RLC Load  LConnTagsString=A|B|C  Configuration=Y (grounded)  NominalVoltage=300e3  Vabc=[1e3 1e3 1e3]  Vabcp=[1e3 1e3 1e3]  NominalFrequency=60  UnbalancedPower=off  ActivePower=0  InductivePower=0  CapacitivePower=2800e6  Pabc=[10e3 9e3 11e3]  QLabc=[100 90 110]  QCabc=[100 90 110]  Pabcp=[10e3 9e3 11e3]  QLabcp=[100 90 110]  QCabcp=[100 90 110]  Measurements=None  LoadType=constant Z
  4200 MW : spsThreePhaseDynamicLoadLib/Three-Phase Dynamic Load  NominalVoltage=[ 20e3 60 ]  ActiveReactivePowers=[4200e6 5.11e-8]  PositiveSequence=[0.994 -11.8]  ExternalControl=off  NpNq=[1.3 2]  TimeConstants="[0  0  0  0]"  MinimumVoltage=0.7  Tfilter=1e-4  LoadFlowParameters=[4,0,0,0,0]
      settings: LibrarySourceBlock=|
      | sps_lib/Passives/Three-Phase
      | Dynamic Load
  4500 MVA 20kV 3780MW : spsAsynchronousMachinepuUnitsLib/Asynchronous Machine pu Units  RotorType=Squirrel-cage  PresetModel=No  MechanicalLoad=Torque Tm  ShowDetailedParameters=on  ReferenceFrame=Rotor  Units=pu  MeasurementBus=off  NominalParameters=[4500e6 20e3 60]  VoltageRatio=1  Stator=[0.01117 0.04832]  Rotor=[0.006 0.04832]  Cage1=[0.01909 0.0397]  Cage2=[0.01909 0.0397]  Lm=2.424  Mechanical="[1  0   2]"  PolePairs=2  InitialConditions=[0.00523668 0 0.941796 0.941796 0.941796 -125.733 -245.733 -5.73298]  SimulateSaturation=off  Saturation="[0.212,0.4201,0.8125,1.0979,1.4799,2.2457,3.2586,4.5763,6.4763 ;   0.5,0.7,0.9,1,1.1,1.2 ,1.3,1.4,1.5]"  LoadFlowParameters=0  TsPowergui=0  TsBlock=-1  IterativeModel=Trapezoidal non iterative  IterativeDiscreteModel=Trapezoidal non iterative  Pmec=3780e6
      settings: LibrarySourceBlock=|
      | sps_lib/Electrical Machines/Asynchronous Machine
      | pu Units
  7500 MW : spsThreePhaseParallelRLCLoadLib/Three-Phase Parallel RLC Load  LConnTagsString=A|B|C  Configuration=Y (grounded)  NominalVoltage=20e3  Vabc=[1e3 1e3 1e3]  Vabcp=[1e3 1e3 1e3]  NominalFrequency=60  UnbalancedPower=off  ActivePower=7500e6  InductivePower=0  CapacitivePower=0  Pabc=[10e3 9e3 11e3]  QLabc=[100 90 110]  QCabc=[100 90 110]  Pabcp=[10e3 9e3 11e3]  QLabcp=[100 90 110]  QCabcp=[100 90 110]  Measurements=None  LoadType=constant Z
  Constant : Constant  Value=0.84021
  Load Flow Bus1 : spsLoadFlowBusLib/Load Flow Bus  LConnTagsString=a  Phases=single  Connectors=on one side  ID=BUS_27  Vbase=20e3  Vref=1  Vangle=0  VLF=1  VLFb=1  VLFc=1  angleLF=0  angleLFb=0  angleLFc=0
  Load Flow Bus4 : spsLoadFlowBusLib/Load Flow Bus  LConnTagsString=a  Phases=single  Connectors=on one side  ID=BUS_26  Vbase=300e3  Vref=1  Vangle=0  VLF=1  VLFb=1  VLFc=1  angleLF=0  angleLFb=0  angleLFc=0
  Terminator : Terminator
  Terminator1 : Terminator
  A : PMIOPort  Side=Left
  B : PMIOPort  Port=2  Side=Left
  C : PMIOPort  Port=3  Side=Left
  wires:
  Constant/1 -> 4500 MVA 20kV 3780MW/1
  4500 MVA 20kV 3780MW/1 -> Terminator1/1
  4200 MW/1 -> Terminator/1
  connections:
  4500 MVA 20kV 3780MW/LConn3 -- 1.8 Mvar/LConn3 -- 7500 MW/LConn3 -- 4200 MW/LConn3 -- "15800 MVA 300KV :20KV Transformer "/RConn3
  "19000 MVA 650KV :300KV Transformer "/RConn1 -- 2800 Mvar/LConn1 -- Load Flow Bus4/LConn1 -- "15800 MVA 300KV :20KV Transformer "/LConn1
  "15800 MVA 300KV :20KV Transformer "/LConn3 -- 2800 Mvar/LConn3 -- "19000 MVA 650KV :300KV Transformer "/RConn3
  4500 MVA 20kV 3780MW/LConn1 -- 1.8 Mvar/LConn1 -- Load Flow Bus1/LConn1 -- "15800 MVA 300KV :20KV Transformer "/RConn1 -- 4200 MW/LConn1 -- 7500 MW/LConn1
  "15800 MVA 300KV :20KV Transformer "/RConn2 -- 7500 MW/LConn2 -- 4500 MVA 20kV 3780MW/LConn2 -- 1.8 Mvar/LConn2 -- 4200 MW/LConn2
  "19000 MVA 650KV :300KV Transformer "/RConn2 -- 2800 Mvar/LConn2 -- "15800 MVA 300KV :20KV Transformer "/LConn2
  "19000 MVA 650KV :300KV Transformer "/LConn2 -- B/RConn1
  "19000 MVA 650KV :300KV Transformer "/LConn1 -- A/RConn1
  "19000 MVA 650KV :300KV Transformer "/LConn3 -- C/RConn1
